simulink model "gov_extended"  (R2020a)
settings: Solver=VariableStepAuto  StartTime=0.0  StopTime=10.0  RelTol=1e-3
values from neighbouring files (symbols this model uses):
  sigma = 0.5    [main.m]
  target = 0.97    [main.m]
  Tf = 0.5    [main.m]
  Tg = 0.1    [main.m]
  To = 0.01    [main.m]
  Tp = 0.01    [main.m]
  tx = 0.4    [main.m]
  VAT = 0.07    [main.m]
settings Model: Creator=erlended  LastModifiedBy=erlended

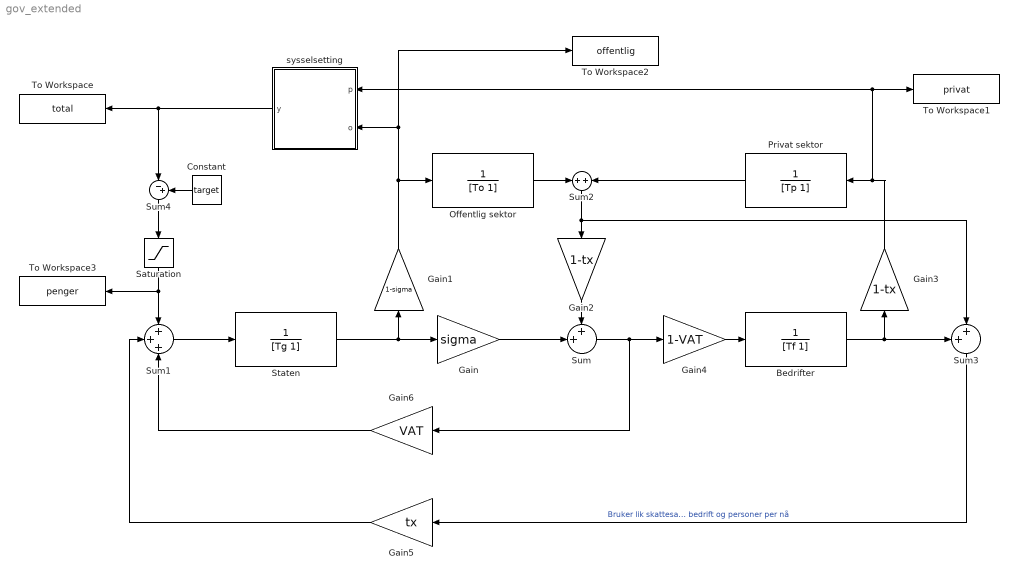
== system gov_extended ==
  Bedrifter : TransferFcn  Denominator=[Tf 1]
  Constant : Constant  Value=target
  Gain : Gain  Gain=sigma
  Gain1 : Gain  Gain=1-sigma
  Gain2 : Gain  Gain=1-tx
  Gain3 : Gain  Gain=1-tx
  Gain4 : Gain  Gain=1-VAT
  Gain5 : Gain  Gain=tx
  Gain6 : Gain  Gain=VAT
  Offentlig sektor : TransferFcn  Denominator=[To 1]
  Privat sektor : TransferFcn  Denominator=[Tp 1]
  Saturation : Saturate  UpperLimit=1  LowerLimit=-1
  Staten : TransferFcn  Denominator=[Tg 1]
  Sum : Sum  Inputs=++|
  Sum1 : Sum  Inputs=+++
  Sum2 : Sum  Inputs=+|+
  Sum3 : Sum  Inputs=++|
  Sum4 : Sum  Inputs=|-+
  To Workspace : ToWorkspace  VariableName=total  SaveFormat=Timeseries  SampleTime=-1
  To Workspace1 : ToWorkspace  VariableName=privat  SaveFormat=Timeseries  SampleTime=-1
  To Workspace2 : ToWorkspace  VariableName=offentlig  SaveFormat=Timeseries  SampleTime=-1
  To Workspace3 : ToWorkspace  VariableName=penger  SaveFormat=Timeseries  SampleTime=-1
  sysselsetting : MATLAB Function  TreatAsAtomicUnit=on
  wires:
  Staten/1 -> Gain/1, Gain1/1
  Sum/1 -> Gain6/1, Gain4/1
  Gain1/1 -> Offentlig sektor/1, To Workspace2/1, sysselsetting/2(o)
  Gain/1 -> Sum/2
  Privat sektor/1 -> Sum2/2
  Sum2/1 -> Gain2/1, Sum3/2
  Offentlig sektor/1 -> Sum2/1
  Sum1/1 -> Staten/1
  Gain4/1 -> Bedrifter/1
  Gain6/1 -> Sum1/3
  sysselsetting/1(y) -> Sum4/1, To Workspace/1
  Bedrifter/1 -> Sum3/1, Gain3/1
  Sum3/1 -> Gain5/1  "Bruker lik skattesats på bedrift og personer per nå"
  Gain5/1 -> Sum1/2
  Gain2/1 -> Sum/1
  Constant/1 -> Sum4/2
  Sum4/1 -> Saturation/1
  Saturation/1 -> To Workspace3/1, Sum1/1
  Gain3/1 -> To Workspace1/1, sysselsetting/1(p), Privat sektor/1

== matlab function gov_extended/sysselsetting ==
  data: p input; o input; y output
function  y= fcn(p, o)
salary = 1; 
employment = (o+p)/salary;

u = employment;

y = u;
